simulink model "MLIB_Neg_BAM"  (Simulink 7.3)
settings: Solver=ode45  StartTime=0.0  StopTime=10.0  RelTol=1e-3
settings Model: Creator=RE004C  LastModifiedBy=RE004C
settings HardwareCC: ProdIntDivRoundTo=Zero  ProdEndianess=BigEndian  ProdHWDeviceType=Freescale->32-bit PowerPC

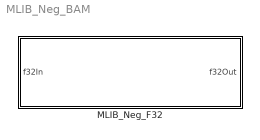
== system MLIB_Neg_BAM ==
  MLIB_Neg_F32 : Subsystem  mask(MLIB_Neg_F32){}
      mask help: Bit accurate model for negative value of input value. All parameters as well as input and output are 32bit integers.
      mask init:
      | pos = get_param(gcb, 'Position');width = pos(3) - pos(1); height = pos(4) - pos(2);tX=width/2;tY=height*0.9;
      mask Display: color('black');port_label('input',1,'f32In');port_label('output',1,'f32Out');color('black');disp('MLIB_Neg_F32');color('blue');text(tX,tY, 'BAM', 'horizontalAlignment', 'center');

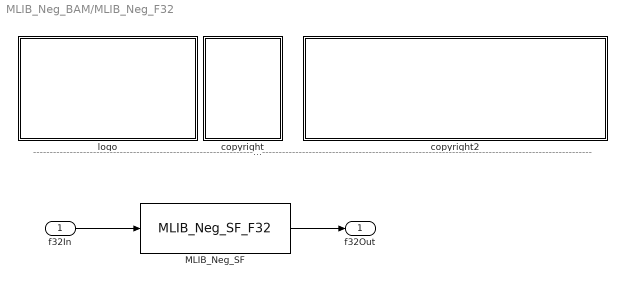
== system MLIB_Neg_BAM/MLIB_Neg_F32 ==
  note: ---------------------------------------------------------------------------------------------------------------------------------------------------------------------------------------------------
  f32In : Inport  OutDataType=fixdt(1, 16)  OutScaling=2^0
  MLIB_Neg_SF : S-Function  FunctionName=MLIB_Neg_SF_F32  EnableBusSupport=off
  copyright : Subsystem
      mask Display: text(10,90,'FILE:');text(10,75,'DESRIPTION:')text(10,60,'COPYRIGHT:')text(10,45,'VERSION:')text(10,30,'DATE:')
  copyright2 : Subsystem
      mask Display: text(10,90,'MLIB_Neg_BAM_F32.mdl');text(10,75,'Sum of two input values.');text(10,60,'Freescale')text(10,45,'0.1');text(10,30,'20-Jan-2012');
  logo : Subsystem
      mask Display: image(imread('logo.jpg'))
  f32Out : Outport  OutDataType=fixdt(1, 16)  OutScaling=2^0
  wires:
  f32In/1 -> MLIB_Neg_SF/1
  MLIB_Neg_SF/1 -> f32Out/1

== system MLIB_Neg_BAM/MLIB_Neg_F32/copyright ==

== system MLIB_Neg_BAM/MLIB_Neg_F32/copyright2 ==

== system MLIB_Neg_BAM/MLIB_Neg_F32/logo ==
